simulink model "output_observer_VTOL_sim"  (R2016b)
settings: Solver=ode45  StartTime=0.0  StopTime=200  RelTol=1e-3  EnableMultiTasking=on
InitFcn:
  | param
undefined symbols (not defined in the file or in its folder): drawVTOL, P, SSctrl_output_observer_fb
settings Model: Creator=beard  LastModifiedBy=jesse
settings DataIOCC: LimitDataPoints=on  SaveFormat=Array  SignalLoggingSaveFormat=ModelDataLogs
settings OptimizationCC: ExpressionDepthLimit=2147483647  InitFltsAndDblsToZero=on  LifeSpan=inf
settings DebuggingCC: UnderspecifiedInitializationDetection=Classic  MergeDetectMultiDrivingBlocksExec=none  SolverPrmCheckMsg=warning  FcnCallInpInsideContextMsg=warning  StateNameClashWarn=warning  SFUnexpectedBacktrackingDiag=warning  SFNoUnconditionalDefaultTransitionDiag=warning  SFExecutionAtInitializationDiag=none
settings HardwareCC: ProdBitPerPointer=32  ProdBitPerSizeT=32  ProdBitPerPtrDiffT=32  ProdLargestAtomicFloat=None  ProdIntDivRoundTo=Undefined  ProdEndianess=Unspecified  ProdWordSize=32  ProdHWDeviceType=32-bit Generic
settings ModelReferenceCC: PropagateSignalLabelsOutOfModel=off
settings GRTTargetCC: TargetLangStandard=C89/C90 (ANSI)  GeneratePreprocessorConditionals=Disable all  CombineOutputUpdateFcns=off  GRTInterface=on
settings ConfigComp: CovMetricSettings=dw  CovHtmlReporting=on  CovSaveCumulativeToWorkspaceVar=on  CovSaveSingleToWorkspaceVar=on  CovExternalEMLEnable=off

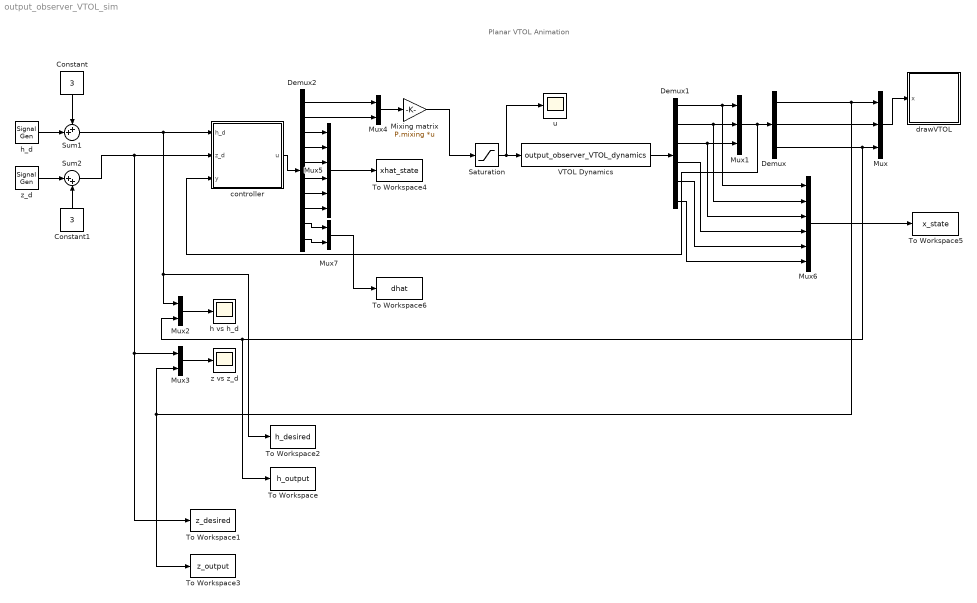
== system output_observer_VTOL_sim ==
  note: Planar VTOL Animation
  Constant : Constant  Value=3
  Constant1 : Constant  Value=3
  Demux : Demux  Outputs=3
  Demux1 : Demux  Outputs=6
  Demux2 : Demux  Outputs=10
  Mixing matrix : Gain  Gain=P.mixing  Multiplication=Matrix(K*u)
  Mux : Mux  Inputs=3
  Mux1 : Mux  Inputs=3
  Mux{2..4,7} (4 alike) : Mux  Inputs=2
  Mux5 : Mux  Inputs=6
  Mux6 : Mux  Inputs=6
  Saturation : Saturate  UpperLimit=P.fmax  LowerLimit=0
  Sum1 : Sum  Inputs=++|
  Sum2 : Sum  Inputs=|++
  To Workspace : ToWorkspace  VariableName=h_output  SaveFormat=Structure With Time  SampleTime=-1
  To Workspace1 : ToWorkspace  VariableName=z_desired  SaveFormat=Structure With Time  SampleTime=-1
  To Workspace2 : ToWorkspace  VariableName=h_desired  SaveFormat=Structure With Time  SampleTime=-1
  To Workspace3 : ToWorkspace  VariableName=z_output  SaveFormat=Structure With Time  SampleTime=-1
  To Workspace4 : ToWorkspace  VariableName=xhat_state  SaveFormat=Structure With Time  SampleTime=-1
  To Workspace5 : ToWorkspace  VariableName=x_state  SaveFormat=Structure With Time  SampleTime=-1
  To Workspace6 : ToWorkspace  VariableName=dhat  SaveFormat=Structure With Time  SampleTime=-1
  VTOL Dynamics : S-Function  FunctionName=output_observer_VTOL_dynamics  Parameters=AP  SFunctionDeploymentMode=off  EnableBusSupport=off
  controller : Subsystem
  drawVTOL : Subsystem
      mask Display: image(imread('tv.jpg'))
  h vs h_d : Scope
  h_d : SignalGenerator  WaveForm=square  Amplitude=2.5  Frequency=.02
  u : Scope
  z vs z_d : Scope
  z_d : SignalGenerator  WaveForm=square  Amplitude=2.5  Frequency=.016
  wires:
  Constant/1 -> Sum1/1
  h_d/1 -> Sum1/2
  Sum2/1 -> controller/2(z_d), Mux3/1, To Workspace1/1
  z_d/1 -> Sum2/1
  Constant1/1 -> Sum2/2
  Saturation/1 -> u/1, VTOL Dynamics/1
  Mixing matrix/1 -> Saturation/1
  Sum1/1 -> controller/1(h_d), Mux2/1, To Workspace2/1
  Mux/1 -> drawVTOL/1(x)
  Mux2/1 -> h vs h_d/1
  Mux3/1 -> z vs z_d/1
  Demux/1 -> Mux3/2, To Workspace3/1, Mux/1
  Demux/2 -> Mux/2
  Demux/3 -> To Workspace/1, Mux2/2, Mux/3
  Demux1/1 -> Mux6/1, Mux1/1
  Demux1/2 -> Mux6/2, Mux1/2
  Demux1/3 -> Mux6/3, Mux1/3
  VTOL Dynamics/1 -> Demux1/1
  Mux1/1 -> controller/3(y), Demux/1
  controller/1(u) -> Demux2/1
  Mux4/1 -> Mixing matrix/1
  Demux2/1 -> Mux4/1
  Demux2/2 -> Mux4/2
  Demux2/3 -> Mux5/1
  Demux2/4 -> Mux5/2
  Demux2/5 -> Mux5/3
  Demux2/6 -> Mux5/4
  Demux2/7 -> Mux5/5
  Demux2/8 -> Mux5/6
  Mux5/1 -> To Workspace4/1
  Demux1/4 -> Mux6/4
  Demux1/5 -> Mux6/5
  Demux1/6 -> Mux6/6
  Mux6/1 -> To Workspace5/1
  Demux2/9 -> Mux7/1
  Demux2/10 -> Mux7/2
  Mux7/1 -> To Workspace6/1

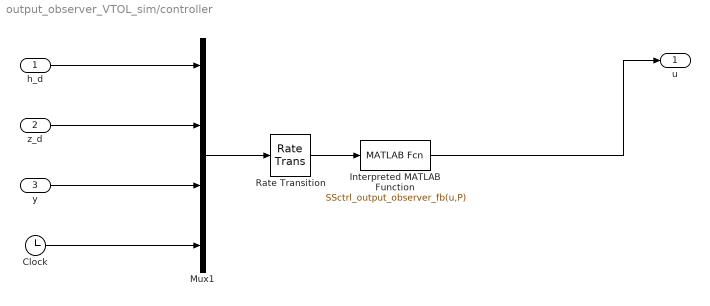
== system output_observer_VTOL_sim/controller ==
  h_d : Inport
  z_d : Inport  Port=2
  y : Inport  Port=3
  Clock : Clock
  Interpreted MATLAB Function : MATLABFcn  MATLABFcn=SSctrl_output_observer_fb(u,P)  OutputDimensions=10
  Mux1 : Mux
  Rate Transition : RateTransition  OutPortSampleTime=P.Ts
  u : Outport
  wires:
  Mux1/1 -> Rate Transition/1
  h_d/1 -> Mux1/1
  Clock/1 -> Mux1/4
  Rate Transition/1 -> Interpreted MATLAB Function/1
  y/1 -> Mux1/3
  z_d/1 -> Mux1/2
  Interpreted MATLAB Function/1 -> u/1

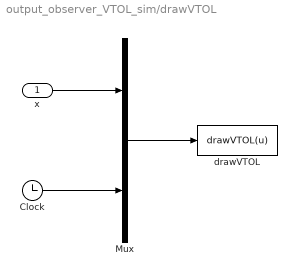
== system output_observer_VTOL_sim/drawVTOL ==
  x : Inport
  Clock : Clock
  Mux : Mux  Inputs=2
  drawVTOL : MATLABFcn  MATLABFcn=drawVTOL(u)  OutputDimensions=0  SampleTime=0.1
  wires:
  Mux/1 -> drawVTOL/1
  x/1 -> Mux/1
  Clock/1 -> Mux/2
